simulink model "Mod1"  (R2018b)
settings: Solver=ode3  StartTime=0.0  StopTime=10  FixedStep=Ts  RelTol=1e-3
undefined symbols (not defined in the file): DiscIntNeverNeededParam, E_nom, f_nom, I_nom, p, R_s, sigbuilder_block, Ts, U_nom, X_d, X_q
libraries: nesl_utility x13, fl_lib x6, pe_lib x5, powerlib_meascontrol x1, elec_lib x1
settings Model: DataDictionary=Data_mod.sldd  Creator=EwgenV  LastModifiedBy=User
settings DebuggingCC: LibraryContextMissingDiagnostic=none
settings SFSimCC: SimUseLocalCustomCode=off
settings RTWCC: RTWUseLocalCustomCode=off

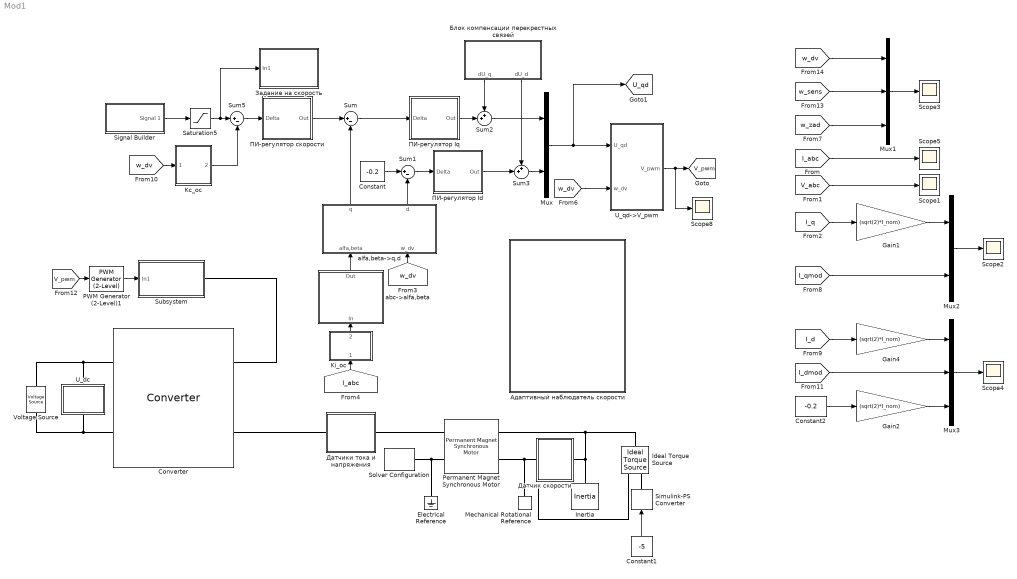
== system Mod1 ==
  Constant : Constant  Value=-0.2
  Constant1 : Constant  Value=-5
  Constant2 : Constant  Value=-0.2
  Converter : pe_lib/Semiconductors/Converter  device_type=2  Vf=0.8 V  Ron=0.001 Ohm  Rds=0.001 Ohm  Goff=1e-6 1/Ohm  Vth=6 V  Vgt=1 V  Vgt_off=-1 V  Ih=1 A  diode_param=2  diode_Vf=0.8 V  diode_Ron=0.0001 Ohm  diode_Goff=1e-5 1/Ohm  diode_C=50 nF  diode_iRM=-235 A  diode_iF=300 A  diode_idot=-50 A/us  diode_trr_param=1  diode_trr_factor=3  diode_trr=15 us  diode_Qrr=1.5e+3 s*uA  snubber_type=0  Rs=0.1 Ohm  Cs=1e-7 F
      settings: SourceProductName=Simscape Electrical  SourceProductBaseCode=PS
  Electrical Reference : fl_lib/Electrical/Electrical Elements/Electrical Reference
  Gain1 : Gain  Gain=(sqrt(2)*I_nom)
  Gain2 : Gain  Gain=(sqrt(2)*I_nom)
  Gain4 : Gain  Gain=(sqrt(2)*I_nom)
  Ideal Torque Source : fl_lib/Mechanical/Mechanical Sources/Ideal Torque Source
  Inertia : fl_lib/Mechanical/Rotational Elements/Inertia  inertia=0.15 kg*m^2  w_specify=off  w_priority=High  w=0 rad/s  w_nominal_specify=off  w_nominal_unit=rad/s  w_nominal_value=1  t_specify=off  t_priority=None  t=0 N*m  t_nominal_specify=off  t_nominal_unit=N*m  t_nominal_value=1
  Kc_oc : Subsystem
  Ki_oc : Subsystem
  Mechanical Rotational Reference : fl_lib/Mechanical/Rotational Elements/Mechanical Rotational Reference
  Mux : Mux  Inputs=2
  Mux1 : Mux  Inputs=3
  Mux2 : Mux  Inputs=2
  Mux3 : Mux  Inputs=3
  PWM Generator (2-Level)1 : powerlib_meascontrol/Pulse & Signal Generators/PWM Generator (2-Level)  ModulatorType=Three-phase bridge (6 pulses)  ModulatorMode=Unsynchronized  Fc=12000  Pc=90  nF=27  MinMax="[ -1  1 ]"  SamplingTechnique=Natural  ModulatingSignals=off  m=0.8  Freq=60  Phase=0  Ts=Ts  ShowCarrierOutport=off
  Permanent Magnet Synchronous Motor : pe_lib/Machines/Permanent Magnet Rotor/Permanent Magnet Synchronous Motor  nPolePairs=5  pmflux_param=1  pm_flux_linkage=E_nom/(2*pi*f_nom) Wb  torque_constant=0.18 N*m/A  back_emf_constant=0.18 V/(rad/s)  stator_param=1  Ld=X_d/(2*pi*f_nom) H  Lq=X_q/(2*pi*f_nom) H  L0=X_q/(2*pi*f_nom) H  Ls=X_q/(2*pi*f_nom) H  Lm=0 H  Ms=0.0001 H  Rs=R_s Ohm  zero_sequence=pe.enum.park.zerosequence.include  J=0.05 kg*m^2  lam=0.000 N*m/(rad/s)  axes_param=pe.enum.rotorangle.daxis  i_d_specify=off  i_d_priority=None  i_d=0 A  i_d_nominal_specify=off  i_d_nominal_unit=A  i_d_nominal_value=1  i_q_specify=off  i_q_priority=None  i_q=0 A  i_q_nominal_specify=off  i_q_nominal_unit=A  i_q_nominal_value=1  torque_specify=on  torque_priority=None  torque=0 N*m  torque_nominal_specify=off  torque_nominal_unit=N*m  torque_nominal_value=1  angular_velocity_specify=off  angular_velocity_priority=High  angular_velocity=0 rpm  angular_velocity_nominal_specify=off  angular_velocity_nominal_unit=rpm  angular_velocity_nominal_value=1  angular_position_specify=off  angular_position_priority=High  angular_position=0 deg  angular_position_nominal_specify=off  angular_position_nominal_unit=deg  angular_position_nominal_value=1
      settings: SourceProductName=Simscape Electrical  SourceProductBaseCode=PS
  Saturation5 : Saturate  UpperLimit=1  LowerLimit=-1
  Scope{1..5,8} (6 alike) : Scope
  Signal Builder : Subsystem  Tag=STV Subsys  LoadFcn=sigbuilder_block('load');  StartFcn=sigbuilder_block('start');  StopFcn=sigbuilder_block('stop');  ClipboardFcn=sigbuilder_block('clipboard');  mask(Sigbuilder block){tuvar=[0:10]}
      mask help: Simulink:masks:SigbuilderBlock_MD
      mask init:
      | if ~strcmp(get_param(bdroot(gcbh),'SimulationStatus'),'stopped') tuvar = sigbuilder_block('maskInit'); end
      settings: CopyFcn=sigbuilder_block('copy');  DeleteFcn=sigbuilder_block('delete');  ModelCloseFcn=sigbuilder_block('modelClose');  PreSaveFcn=sigbuilder_block('preSave');  PauseFcn=sigbuilder_block('pause');  ContinueFcn=sigbuilder_block('continue');  NameChangeFcn=sigbuilder_block('namechange');  OpenFcn=sigbuilder_block('open',[437.6 199.2 550.4 400 ]);  CloseFcn=sigbuilder_block('close');
      mask Display: plot(0, 0, 100, 100,[2, 2, 32, 32, 2], [68, 8, 8, 68, 68],[32, 2], [38, 38], [32, 19, 2],[53, 60, 44], [32, 17, 17, 2],[16, 16, 31, 31]);txt = getActiveGroup(gcbh);text(2, 100, txt,'verticalAlignment', 'top');
  Simulink-PS Converter : nesl_utility/Simulink-PS Converter  PhysicalDomain=network_engine_domain  SubClassName=ps_input  LeftPortType=input  RightPortType=output  PseudoPeriodic=off  Frequencies=[]  NoiseDistribution=none  NoiseParameters=[]  Unit=1  AffineConversion=off  FilteringAndDerivatives=provide  SimscapeFilterOrder=1  InputFilterTimeConstant=0.001  UdotUserProvided=0
  Solver Configuration : nesl_utility/Solver Configuration  PhysicalDomain=network_engine_domain  SubClassName=solver  LeftPortType=input  RightPortType=generic  Tones=[]  Harmonics=[]  SimulateNoise=off  Profile=off  UseLocalSampling=off  EnableSwitchedLinearOptims=on  FrequencyDomain=off  UseCCode=off  RelTol=0.001  AbsTol=1e-06  MinStep=1e-09  ToWorkspace=off  RevertToSquareIcSolve=off  NumHomotopyIterations=100  PhasorMode=off  PhasorModeNumHarmonics=1  DoDC=off  ResidualTolerance=1e-09  UseLocalSolver=on  LocalSolverChoice=NE_BACKWARD_EULER_ADVANCER  LocalSolverSampleTime=Ts  DoFixedCost=on  MaxNonlinIter=3  MaxModeIter=2  LinearAlgebra=Sparse  EquationFormulation=NE_TIME_EF  DelaysMemoryBudget=1024  AutomaticFiltering=on  FilteringTimeConstant=0.001  PartitionStorageMethod=AS_NEEDED  PartitionMemoryBudget=1024
  Subsystem : Subsystem
  Sum : Sum  Inputs=|+-
  Sum1 : Sum  Inputs=|+-
  Sum2 : Sum  Inputs=++|
  Sum3 : Sum  Inputs=++|
  Sum5 : Sum  Inputs=|+-
  U_dc : Subsystem
  U_qd->V_pwm : Subsystem
  Voltage Source : elec_lib/Sources/Voltage Source  dc_voltage=540 V  ac_voltage=0 V  ac_shift=0 rad  ac_frequency=0 Hz  noise_mode=0  PSD=0 V^2/Hz  repeatability=1  auto_seed=3499211588  user_seed=0  sample_time=1e-3 s  i_specify=off  i_priority=None  i=0 A  i_nominal_specify=off  i_nominal_unit=A  i_nominal_value=1  v_specify=off  v_priority=None  v=0 V  v_nominal_specify=off  v_nominal_unit=V  v_nominal_value=1
      settings: SourceProductName=Simscape Electronics  SourceProductBaseCode=SN
  abc->alfa,beta : Subsystem
  alfa,beta->q,d : Subsystem
  Адаптивный наблюдатель скорости : Subsystem
  Блок компенсации перекрестных связей : Subsystem
  Датчик скорости : Subsystem
  Датчики тока и напряжения : Subsystem
  Задание на скорость : Subsystem
  ПИ-регулятор Id : Subsystem  mask{Kp=0.5, Ki=1, Max=1, Min=-1}
      mask prompts: Kp "Пропорциональный коэффициент"; Ki "Интегральный коэффициент"; Max "Максимум выхода ПИ-регулятора"; Min "Минимум выхода ПИ-регулятора"
      mask DialogControl DescGroupVar Prompt: ПИ-регулятор
      mask DialogControl ParameterGroupVar Prompt: Параметры
  ПИ-регулятор Iq : Subsystem  mask{Kp=0.5, Ki=1, Max=1, Min=-1}
      mask prompts: Kp "Пропорциональный коэффициент"; Ki "Интегральный коэффициент"; Max "Максимум выхода ПИ-регулятора"; Min "Минимум выхода ПИ-регулятора"
      mask DialogControl DescGroupVar Prompt: ПИ-регулятор
      mask DialogControl ParameterGroupVar Prompt: Параметры
  ПИ-регулятор скорости : Subsystem  mask{Kp=50, Ki=10, Max=1.5, Min=-1.5}
      mask prompts: Kp "Пропорциональный коэффициент"; Ki "Интегральный коэффициент"; Max "Максимум выхода ПИ-регулятора"; Min "Минимум выхода ПИ-регулятора"
      mask DialogControl DescGroupVar Prompt: ПИ-регулятор
      mask DialogControl ParameterGroupVar Prompt: Параметры
  tag scope: U_qd=global, V_pwm=global
  wires:
  [I_abc] -> Scope5/1
  [V_abc] -> Scope1/1
  abc->alfa,beta/1(Out) -> alfa,beta->q,d/1(alfa,beta)
  [w_dv] -> alfa,beta->q,d/2(w_dv)
  Sum5/1 -> ПИ-регулятор скорости/1(Delta)
  ПИ-регулятор Iq/1(Out) -> Sum2/2
  ПИ-регулятор Id/1(Out) -> Sum3/2
  Saturation5/1 -> Задание на скорость/1(In1), Sum5/1
  Sum/1 -> ПИ-регулятор Iq/1(Delta)
  Sum1/1 -> ПИ-регулятор Id/1(Delta)
  Mux/1 -> [U_qd], U_qd->V_pwm/1(U_qd)
  [w_dv] -> U_qd->V_pwm/2(w_dv)
  U_qd->V_pwm/1(V_pwm) -> Scope8/1, [V_pwm]
  [w_dv] -> Kc_oc/1(1)
  Kc_oc/1(2) -> Sum5/2
  [I_abc] -> Ki_oc/1(1)
  Ki_oc/1(2) -> abc->alfa,beta/1(In)
  Sum2/1 -> Mux/1
  Sum3/1 -> Mux/2
  alfa,beta->q,d/1("q ") -> Sum/2
  alfa,beta->q,d/2(d) -> Sum1/2
  Constant/1 -> Sum1/1
  Блок компенсации перекрестных связей/1(dU_q) -> Sum2/1
  Блок компенсации перекрестных связей/2(dU_d) -> Sum3/1
  [w_dv] -> Mux1/1
  Mux1/1 -> Scope3/1
  [w_sens] -> Mux1/2
  [w_zad] -> Mux1/3
  Mux2/1 -> Scope2/1
  [I_q] -> Gain1/1
  [I_qmod] -> Mux2/2
  [I_dmod] -> Mux3/2
  [I_d] -> Gain4/1
  Mux3/1 -> Scope4/1
  Gain4/1 -> Mux3/1
  Gain1/1 -> Mux2/1
  [V_pwm] -> PWM Generator (2-Level)1/1
  PWM Generator (2-Level)1/1 -> Subsystem/1(In1)
  ПИ-регулятор скорости/1(Out) -> Sum/1
  Constant1/1 -> Simulink-PS Converter/1
  Gain2/1 -> Mux3/3
  Constant2/1 -> Gain2/1
  Signal Builder/1(Signal 1) -> Saturation5/1
  connections:
  Electrical Reference/LConn1 -- Solver Configuration/RConn1 -- Permanent Magnet Synchronous Motor/LConn2
  Inertia/LConn1 -- Ideal Torque Source/LConn1 -- Permanent Magnet Synchronous Motor/RConn1 -- Датчик скорости/RConn1
  Mechanical Rotational Reference/LConn1 -- Ideal Torque Source/RConn2 -- Датчик скорости/LConn1 -- Permanent Magnet Synchronous Motor/RConn2
  Датчики тока и напряжения/RConn1 -- Permanent Magnet Synchronous Motor/LConn1
  Simulink-PS Converter/RConn1 -- Ideal Torque Source/RConn1
  Voltage Source/LConn1 -- U_dc/LConn1 -- Converter/RConn1
  Voltage Source/RConn1 -- U_dc/RConn1 -- Converter/RConn2
  Converter/LConn2 -- Датчики тока и напряжения/LConn1
  Subsystem/RConn1 -- Converter/LConn1

== system Mod1/Kc_oc ==
  1 : Inport
  Delay3 : Delay  DelayLength=1  InitialCondition=0
  Gain15 : Gain  Gain=p/(2*pi*f_nom)
  2 : Outport
  wires:
  Delay3/1 -> Gain15/1
  Gain15/1 -> 2/1
  1/1 -> Delay3/1

== system Mod1/Ki_oc ==
  1 : Inport
  Delay1 : Delay  DelayLength=1  InitialCondition=0
  Gain : Gain  Gain=1/(sqrt(2)*I_nom)
  2 : Outport
  wires:
  Delay1/1 -> Gain/1
  1/1 -> Delay1/1
  Gain/1 -> 2/1

== system Mod1/Signal Builder ==
  Demux : Demux  Tag=STV Demux  Outputs=1
  FromWs : FromWorkspace  Tag=STV FromWs  VariableName=tuvar  SampleTime=0
      SigBuilderData=|
      | common.afterFinalStr = 'Extrapolate'
      | common.sampleTime = 0
      | dataSet.timeRange = [0 10]
      | dataSet.name = 'Group 1'
      | sbobj.Groups.Name = 'Group 1'
      | sbobj.Groups.Signals.Name = 'Signal 1'
      | sbobj.Groups.Signals.XData = [0 0.1 1 1.15 2 2.25 4.5 5 5.5 6 8.5 9 9.2 9.2 9.3 10]
      | sbobj.Groups.Signals.YData = [0 0.2 0.2 0.5 0.5 1 1 0 0 -1 -1 0 0 -0.0055 0.2 0.2]
  Signal 1 : Outport  Tag=STV Outport
  wires:
  Demux/1 -> Signal 1/1
  FromWs/1 -> Demux/1

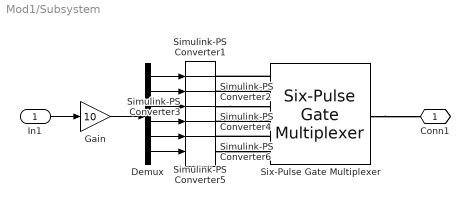
== system Mod1/Subsystem ==
  In1 : Inport
  Demux : Demux  Outputs=6
  Gain : Gain  Gain=10
  Simulink-PS Converter{1..6} (6 alike) : nesl_utility/Simulink-PS Converter  PhysicalDomain=network_engine_domain  SubClassName=ps_input  LeftPortType=input  RightPortType=output  PseudoPeriodic=off  Frequencies=[]  NoiseDistribution=none  NoiseParameters=[]  Unit=1  AffineConversion=off  FilteringAndDerivatives=provide  SimscapeFilterOrder=1  InputFilterTimeConstant=0.001  UdotUserProvided=0
  Six-Pulse Gate Multiplexer : pe_lib/Semiconductors/Six-Pulse Gate Multiplexer  R=0 Ohm
      settings: SourceProductName=Simscape Electrical  SourceProductBaseCode=PS
  Conn1 : PMIOPort  Side=Right
  wires:
  Demux/2 -> Simulink-PS Converter2/1
  Demux/4 -> Simulink-PS Converter4/1
  Demux/3 -> Simulink-PS Converter3/1
  Demux/6 -> Simulink-PS Converter6/1
  Demux/5 -> Simulink-PS Converter5/1
  Demux/1 -> Simulink-PS Converter1/1
  Gain/1 -> Demux/1
  In1/1 -> Gain/1
  connections:
  Six-Pulse Gate Multiplexer/LConn5 -- Simulink-PS Converter5/RConn1
  Six-Pulse Gate Multiplexer/RConn1 -- Conn1/RConn1
  Six-Pulse Gate Multiplexer/LConn4 -- Simulink-PS Converter4/RConn1
  Six-Pulse Gate Multiplexer/LConn1 -- Simulink-PS Converter1/RConn1
  Simulink-PS Converter3/RConn1 -- Six-Pulse Gate Multiplexer/LConn3
  Simulink-PS Converter6/RConn1 -- Six-Pulse Gate Multiplexer/LConn6
  Six-Pulse Gate Multiplexer/LConn2 -- Simulink-PS Converter2/RConn1

== system Mod1/U_dc ==
  PS-Simulink Converter : nesl_utility/PS-Simulink Converter  PhysicalDomain=network_engine_domain  SubClassName=ps_output  LeftPortType=input  RightPortType=output  PseudoPeriodic=off  Frequencies=[]  Unit=1  AffineConversion=off
  Voltage Sensor : fl_lib/Electrical/Electrical Sensors/Voltage Sensor
  "+ " : PMIOPort  Side=Left
  "- " : PMIOPort  Port=2  Side=Right
  tag scope: U_dc=global
  wires:
  PS-Simulink Converter/1 -> [U_dc]
  connections:
  PS-Simulink Converter/LConn1 -- Voltage Sensor/RConn1
  Voltage Sensor/RConn2 -- "- "/RConn1
  Voltage Sensor/LConn1 -- "+ "/RConn1

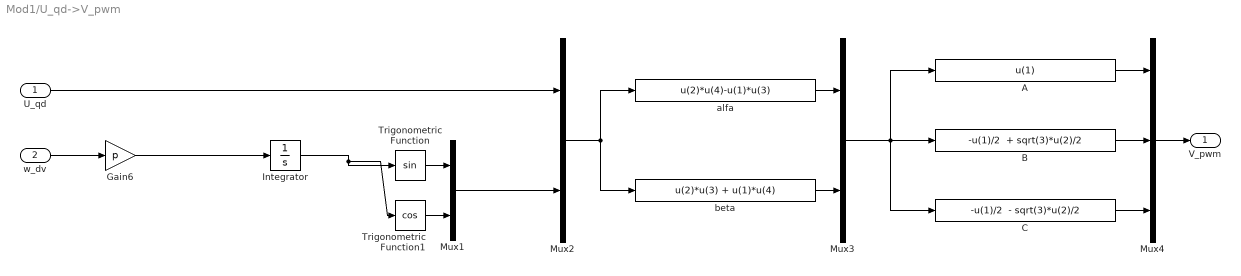
== system Mod1/U_qd->V_pwm ==
  U_qd : Inport
  w_dv : Inport  Port=2
  A : Fcn  Expr=u(1)
  B : Fcn  Expr="-u(1)/2  + sqrt(3)*u(2)/2"
  Gain6 : Gain  Gain=p
  Integrator : Integrator
  Mux1 : Mux  Inputs=2
  Mux2 : Mux  Inputs=2
  Mux3 : Mux  Inputs=2
  Mux4 : Mux  Inputs=3
  Trigonometric Function : Trigonometry
  Trigonometric Function1 : Trigonometry  Operator=cos
  "alfa " : Fcn  Expr=u(2)*u(4)-u(1)*u(3)
  beta : Fcn  Expr=u(2)*u(3) + u(1)*u(4)
  С : Fcn  Expr="-u(1)/2  - sqrt(3)*u(2)/2"
  V_pwm : Outport
  wires:
  beta/1 -> Mux3/2
  "alfa "/1 -> Mux3/1
  Mux1/1 -> Mux2/2
  С/1 -> Mux4/3
  Gain6/1 -> Integrator/1
  Mux2/1 -> beta/1, "alfa "/1
  Mux3/1 -> С/1, B/1, A/1
  Trigonometric Function/1 -> Mux1/1
  A/1 -> Mux4/1
  w_dv/1 -> Gain6/1
  Trigonometric Function1/1 -> Mux1/2
  Mux4/1 -> V_pwm/1
  B/1 -> Mux4/2
  U_qd/1 -> Mux2/1
  Integrator/1 -> Trigonometric Function1/1, Trigonometric Function/1

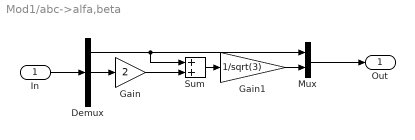
== system Mod1/abc->alfa,beta ==
  In : Inport
  Demux : Demux  Outputs=3
  Gain : Gain  Gain=2
  Gain1 : Gain  Gain=1/sqrt(3)
  Mux : Mux  Inputs=2
  Sum : Sum
  Out : Outport
  wires:
  Gain1/1 -> Mux/2
  Demux/1 -> Sum/1, Mux/1
  Demux/2 -> Gain/1
  Gain/1 -> Sum/2
  Sum/1 -> Gain1/1
  Mux/1 -> Out/1
  In/1 -> Demux/1

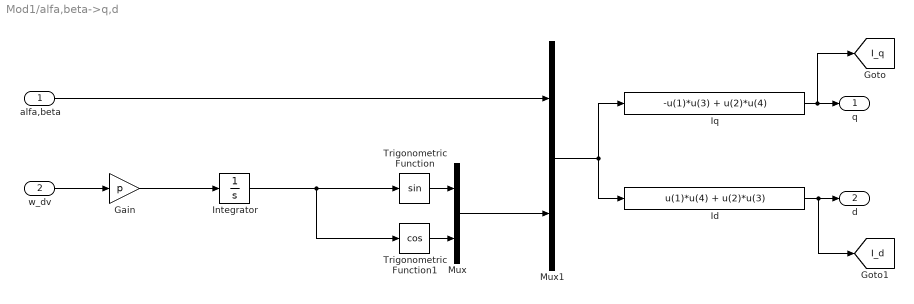
== system Mod1/alfa,beta->q,d ==
  alfa,beta : Inport
  w_dv : Inport  Port=2
  Gain : Gain  Gain=p
  "Id " : Fcn  Expr=u(1)*u(4) + u(2)*u(3)
  Integrator : Integrator
  Iq : Fcn  Expr=-u(1)*u(3) + u(2)*u(4)
  Mux : Mux  Inputs=2
  Mux1 : Mux  Inputs=2
  Trigonometric Function : Trigonometry
  Trigonometric Function1 : Trigonometry  Operator=cos
  "q " : Outport
  d : Outport  Port=2
  tag scope: I_d=global, I_q=global
  wires:
  Mux1/1 -> "Id "/1, Iq/1
  Integrator/1 -> Trigonometric Function/1, Trigonometric Function1/1
  Iq/1 -> [I_q], "q "/1
  Trigonometric Function/1 -> Mux/1
  Trigonometric Function1/1 -> Mux/2
  Mux/1 -> Mux1/2
  Gain/1 -> Integrator/1
  "Id "/1 -> [I_d], d/1
  w_dv/1 -> Gain/1
  alfa,beta/1 -> Mux1/1

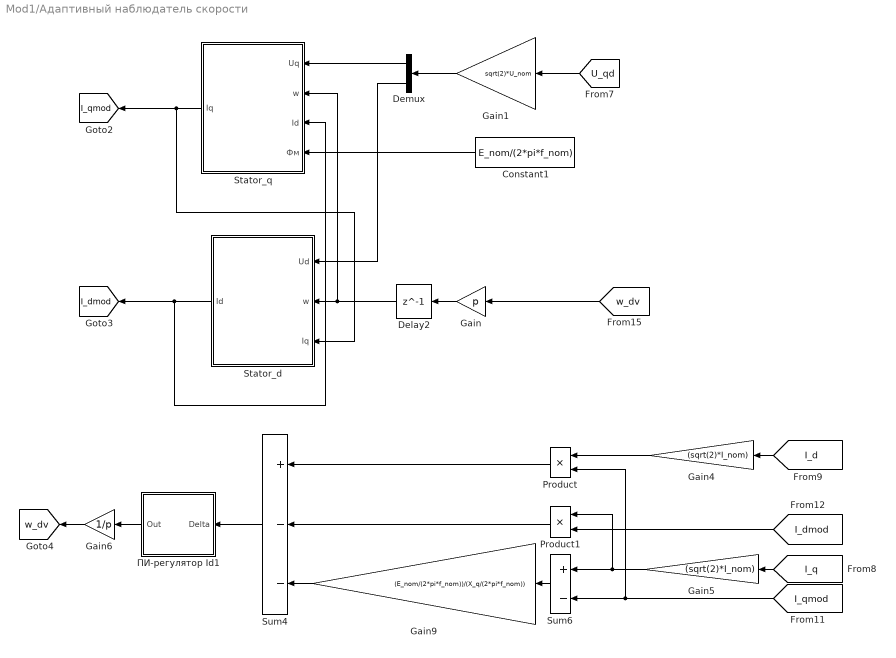
== system Mod1/Адаптивный наблюдатель скорости ==
  Constant1 : Constant  Value=E_nom/(2*pi*f_nom)
  Delay2 : Delay  DelayLength=1  InitialCondition=0
  Demux : Demux  Outputs=2
  Gain : Gain  Gain=p
  Gain1 : Gain  Gain=sqrt(2)*U_nom
  Gain4 : Gain  Gain=(sqrt(2)*I_nom)
  Gain5 : Gain  Gain=(sqrt(2)*I_nom)
  Gain6 : Gain  Gain=1/p
  Gain9 : Gain  Gain=(E_nom/(2*pi*f_nom))/(X_q/(2*pi*f_nom))
  Product : Product
  Product1 : Product
  Stator_d : Subsystem
  Stator_q : Subsystem
  Sum4 : Sum  Inputs=+--
  Sum6 : Sum  Inputs=+-
  ПИ-регулятор Id1 : Subsystem  mask{Kp=0.02, Ki=5, Max=1500, Min=-1500}
      mask prompts: Kp "Пропорциональный коэффициент"; Ki "Интегральный коэффициент"; Max "Максимум выхода ПИ-регулятора"; Min "Минимум выхода ПИ-регулятора"
      mask DialogControl DescGroupVar Prompt: ПИ-регулятор
      mask DialogControl ParameterGroupVar Prompt: Параметры
  tag scope: I_dmod=global, I_qmod=global, w_dv=global
  wires:
  Product1/1 -> Sum4/2
  Sum4/1 -> ПИ-регулятор Id1/1(Delta)
  Constant1/1 -> Stator_q/4(Фм)
  Demux/1 -> Stator_q/1("Uq ")
  Sum6/1 -> Gain9/1
  Gain5/1 -> Product1/1, Sum6/1
  Demux/2 -> Stator_d/1("Ud ")
  Gain1/1 -> Demux/1
  [U_qd] -> Gain1/1
  Stator_d/1(Id) -> [I_dmod], Stator_q/3("Id ")
  Stator_q/1(Iq) -> [I_qmod], Stator_d/3("Iq ")
  Gain6/1 -> [w_dv]
  Gain/1 -> Delay2/1
  [I_dmod] -> Product1/2
  [I_qmod] -> Product/2, Sum6/2
  Delay2/1 -> Stator_q/2("w "), Stator_d/2("w ")
  Gain4/1 -> Product/1
  Gain9/1 -> Sum4/3
  ПИ-регулятор Id1/1(Out) -> Gain6/1
  Product/1 -> Sum4/1
  [I_d] -> Gain4/1
  [I_q] -> Gain5/1
  [w_dv] -> Gain/1

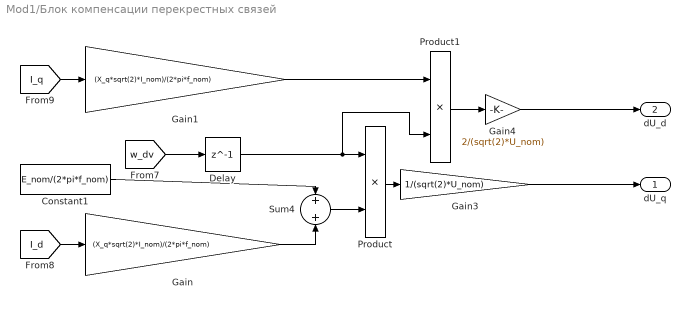
== system Mod1/Блок компенсации перекрестных связей ==
  Constant1 : Constant  Value=E_nom/(2*pi*f_nom)
  Delay : Delay  DelayLength=1  InitialCondition=0
  Gain : Gain  Gain=(X_q*sqrt(2)*I_nom)/(2*pi*f_nom)
  Gain1 : Gain  Gain=(X_q*sqrt(2)*I_nom)/(2*pi*f_nom)
  Gain3 : Gain  Gain=1/(sqrt(2)*U_nom)
  Gain4 : Gain  Gain=2/(sqrt(2)*U_nom)
  Product : Product
  Product1 : Product
  Sum4 : Sum
  dU_q : Outport
  dU_d : Outport  Port=2
  wires:
  Constant1/1 -> Sum4/1
  Delay/1 -> Product1/2, Product/1
  [I_d] -> Gain/1
  [I_q] -> Gain1/1
  Gain/1 -> Sum4/2
  Product/1 -> Gain3/1
  Sum4/1 -> Product/2
  Gain1/1 -> Product1/1
  [w_dv] -> Delay/1
  Product1/1 -> Gain4/1
  Gain3/1 -> dU_q/1
  Gain4/1 -> dU_d/1

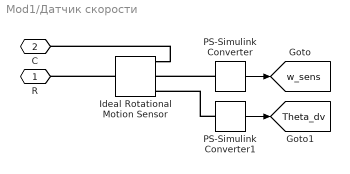
== system Mod1/Датчик скорости ==
  Ideal Rotational Motion Sensor : fl_lib/Mechanical/Mechanical Sensors/Ideal Rotational Motion Sensor  offset=0 rad
  PS-Simulink Converter : nesl_utility/PS-Simulink Converter  PhysicalDomain=network_engine_domain  SubClassName=ps_output  LeftPortType=input  RightPortType=output  PseudoPeriodic=off  Frequencies=[]  Unit=1  AffineConversion=off
  PS-Simulink Converter1 : nesl_utility/PS-Simulink Converter  PhysicalDomain=network_engine_domain  SubClassName=ps_output  LeftPortType=input  RightPortType=output  PseudoPeriodic=off  Frequencies=[]  Unit=1  AffineConversion=off
  R : PMIOPort  Side=Right
  C : PMIOPort  Port=2  Side=Left
  tag scope: Theta_dv=global, w_sens=global
  wires:
  PS-Simulink Converter/1 -> [w_sens]
  PS-Simulink Converter1/1 -> [Theta_dv]
  connections:
  PS-Simulink Converter1/LConn1 -- Ideal Rotational Motion Sensor/RConn3
  PS-Simulink Converter/LConn1 -- Ideal Rotational Motion Sensor/RConn2
  Ideal Rotational Motion Sensor/LConn1 -- R/RConn1
  Ideal Rotational Motion Sensor/RConn1 -- C/RConn1

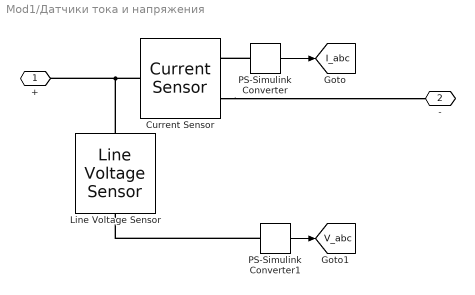
== system Mod1/Датчики тока и напряжения ==
  Current Sensor : pe_lib/Sensors/Current Sensor
      settings: SourceProductName=Simscape Electrical  SourceProductBaseCode=PS
  Line Voltage Sensor : pe_lib/Sensors/Line Voltage Sensor
      settings: SourceProductName=Simscape Electrical  SourceProductBaseCode=PS
  PS-Simulink Converter : nesl_utility/PS-Simulink Converter  PhysicalDomain=network_engine_domain  SubClassName=ps_output  LeftPortType=input  RightPortType=output  PseudoPeriodic=off  Frequencies=[]  Unit=1  AffineConversion=off
  PS-Simulink Converter1 : nesl_utility/PS-Simulink Converter  PhysicalDomain=network_engine_domain  SubClassName=ps_output  LeftPortType=input  RightPortType=output  PseudoPeriodic=off  Frequencies=[]  Unit=1  AffineConversion=off
  + : PMIOPort  Side=Left
  - : PMIOPort  Port=2  Side=Right
  tag scope: I_abc=global, V_abc=global
  wires:
  PS-Simulink Converter/1 -> [I_abc]
  PS-Simulink Converter1/1 -> [V_abc]
  connections:
  Current Sensor/RConn2 -- -/RConn1
  PS-Simulink Converter/LConn1 -- Current Sensor/RConn1
  PS-Simulink Converter1/LConn1 -- Line Voltage Sensor/RConn1
  Line Voltage Sensor/LConn1 -- +/RConn1 -- Current Sensor/LConn1

== system Mod1/Задание на скорость ==
  In1 : Inport
  Gain15 : Gain  Gain=(2*pi*f_nom)/p
  tag scope: w_zad=global
  wires:
  Gain15/1 -> [w_zad]
  In1/1 -> Gain15/1

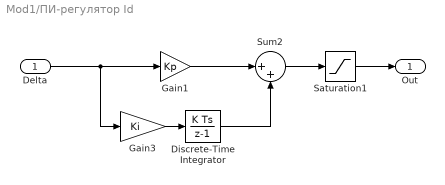
== system Mod1/ПИ-регулятор Id ==
  Delta : Inport
  Discrete-Time Integrator : DiscreteIntegrator  SampleTime=-1  LimitOutput=on  UpperSaturationLimit=Max  LowerSaturationLimit=Min  ICPrevOutput=DiscIntNeverNeededParam  ICPrevScaledInput=DiscIntNeverNeededParam
  Gain1 : Gain  Gain=Kp
  Gain3 : Gain  Gain=Ki
  Saturation1 : Saturate  UpperLimit=Max  LowerLimit=Min
  Sum2 : Sum  Inputs=|++
  Out : Outport
  wires:
  Saturation1/1 -> Out/1
  Sum2/1 -> Saturation1/1
  Discrete-Time Integrator/1 -> Sum2/2
  Delta/1 -> Gain1/1, Gain3/1
  Gain1/1 -> Sum2/1
  Gain3/1 -> Discrete-Time Integrator/1

== system Mod1/ПИ-регулятор Iq ==
  Delta : Inport
  Discrete-Time Integrator : DiscreteIntegrator  SampleTime=-1  LimitOutput=on  UpperSaturationLimit=Max  LowerSaturationLimit=Min  ICPrevOutput=DiscIntNeverNeededParam  ICPrevScaledInput=DiscIntNeverNeededParam
  Gain1 : Gain  Gain=Kp
  Gain3 : Gain  Gain=Ki
  Saturation1 : Saturate  UpperLimit=Max  LowerLimit=Min
  Sum2 : Sum  Inputs=|++
  Out : Outport
  wires:
  Gain3/1 -> Discrete-Time Integrator/1
  Gain1/1 -> Sum2/1
  Delta/1 -> Gain3/1, Gain1/1
  Discrete-Time Integrator/1 -> Sum2/2
  Sum2/1 -> Saturation1/1
  Saturation1/1 -> Out/1

== system Mod1/ПИ-регулятор скорости ==
  Delta : Inport
  Discrete-Time Integrator : DiscreteIntegrator  SampleTime=Ts  LimitOutput=on  UpperSaturationLimit=Max  LowerSaturationLimit=Min  ICPrevOutput=DiscIntNeverNeededParam  ICPrevScaledInput=DiscIntNeverNeededParam
  Gain1 : Gain  Gain=Kp
  Gain3 : Gain  Gain=Ki
  Saturation1 : Saturate  UpperLimit=Max  LowerLimit=Min
  Sum2 : Sum  Inputs=|++
  Out : Outport
  wires:
  Saturation1/1 -> Out/1
  Sum2/1 -> Saturation1/1
  Discrete-Time Integrator/1 -> Sum2/2
  Delta/1 -> Gain1/1, Gain3/1
  Gain3/1 -> Discrete-Time Integrator/1
  Gain1/1 -> Sum2/1

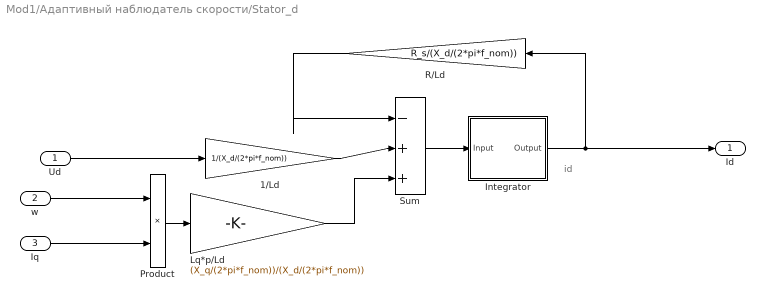
== system Mod1/Адаптивный наблюдатель скорости/Stator_d ==
  note: id
  "Ud " : Inport
  "w " : Inport  Port=2
  "Iq " : Inport  Port=3
  1/Ld : Gain  Gain=1/(X_d/(2*pi*f_nom))
  Integrator : Subsystem
  Lq*p/Ld : Gain  Gain=(X_q/(2*pi*f_nom))/(X_d/(2*pi*f_nom))
  Product : Product
  R/Ld : Gain  Gain=R_s/(X_d/(2*pi*f_nom))
  Sum : Sum  Inputs=|-++
  Id : Outport
  wires:
  "Ud "/1 -> 1/Ld/1
  1/Ld/1 -> Sum/2
  Product/1 -> Lq*p/Ld/1
  Lq*p/Ld/1 -> Sum/3
  "Iq "/1 -> Product/2
  "w "/1 -> Product/1
  Sum/1 -> Integrator/1(Input)
  R/Ld/1 -> Sum/1
  Integrator/1(Output) -> Id/1, R/Ld/1

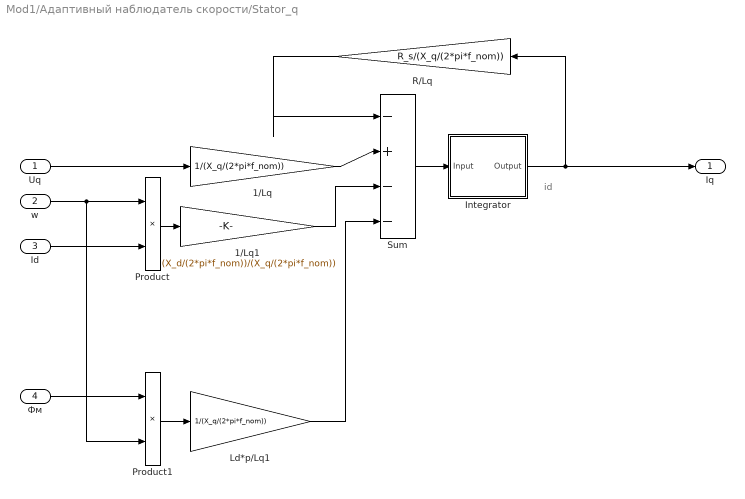
== system Mod1/Адаптивный наблюдатель скорости/Stator_q ==
  note: id
  "Uq " : Inport
  "w " : Inport  Port=2
  "Id " : Inport  Port=3
  Фм : Inport  Port=4
  1/Lq : Gain  Gain=1/(X_q/(2*pi*f_nom))
  1/Lq1 : Gain  Gain=(X_d/(2*pi*f_nom))/(X_q/(2*pi*f_nom))
  Integrator : Subsystem
  Ld*p/Lq1 : Gain  Gain=1/(X_q/(2*pi*f_nom))
  Product : Product
  Product1 : Product
  R/Lq : Gain  Gain=R_s/(X_q/(2*pi*f_nom))
  Sum : Sum  Inputs=|-+--
  Iq : Outport
  wires:
  "Uq "/1 -> 1/Lq/1
  1/Lq/1 -> Sum/2
  Product/1 -> 1/Lq1/1
  1/Lq1/1 -> Sum/3
  "Id "/1 -> Product/2
  "w "/1 -> Product1/2, Product/1
  Sum/1 -> Integrator/1(Input)
  R/Lq/1 -> Sum/1
  Integrator/1(Output) -> R/Lq/1, Iq/1
  Фм/1 -> Product1/1
  Product1/1 -> Ld*p/Lq1/1
  Ld*p/Lq1/1 -> Sum/4

== system Mod1/Адаптивный наблюдатель скорости/ПИ-регулятор Id1 ==
  Delta : Inport
  Discrete-Time Integrator : DiscreteIntegrator  SampleTime=-1  LimitOutput=on  UpperSaturationLimit=Max  LowerSaturationLimit=Min  ICPrevOutput=DiscIntNeverNeededParam  ICPrevScaledInput=DiscIntNeverNeededParam
  Gain1 : Gain  Gain=Kp
  Gain3 : Gain  Gain=Ki
  Saturation1 : Saturate  UpperLimit=Max  LowerLimit=Min
  Sum2 : Sum  Inputs=|++
  Out : Outport
  wires:
  Gain3/1 -> Discrete-Time Integrator/1
  Gain1/1 -> Sum2/1
  Delta/1 -> Gain3/1, Gain1/1
  Discrete-Time Integrator/1 -> Sum2/2
  Sum2/1 -> Saturation1/1
  Saturation1/1 -> Out/1

== system Mod1/Адаптивный наблюдатель скорости/Stator_d/Integrator ==
  Input : Inport
  Delay : Delay  DelayLength=1  InitialCondition=0
  Gain3 : Gain  Gain=Ts
  Sum4 : Sum  Inputs=|++
  Output : Outport
  wires:
  Delay/1 -> Sum4/2
  Input/1 -> Gain3/1
  Sum4/1 -> Output/1, Delay/1
  Gain3/1 -> Sum4/1

== system Mod1/Адаптивный наблюдатель скорости/Stator_q/Integrator ==
  Input : Inport
  Delay : Delay  DelayLength=1  InitialCondition=0
  Gain3 : Gain  Gain=Ts
  Sum4 : Sum  Inputs=|++
  Output : Outport
  wires:
  Delay/1 -> Sum4/2
  Input/1 -> Gain3/1
  Sum4/1 -> Output/1, Delay/1
  Gain3/1 -> Sum4/1
